simulink model "calcparam1cell"  (R2019a)
settings: Solver=VariableStepAuto  StartTime=0.0  StopTime=2335  RelTol=1e-3
values from neighbouring files (symbols this model uses):
  Q = 31.2    [workspace.mat]
undefined symbols (not defined in the file or in its folder): c1, r0, r1, sigbuilder_block, soc_1
settings Model: Creator=sujan  LastModifiedBy=sujan

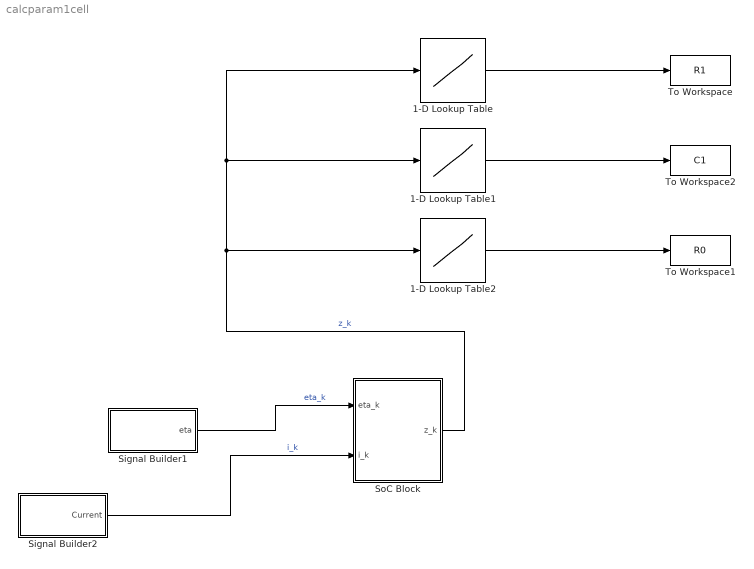
== system calcparam1cell ==
  1-D Lookup Table : Lookup_n-D  NumberOfTableDimensions=1  BreakpointsForDimension1=soc_1.soc_1  Table=r1.r1  InternalRulePriority=Speed  RndMeth=Simplest  InputSameDT=on
  1-D Lookup Table1 : Lookup_n-D  NumberOfTableDimensions=1  BreakpointsForDimension1=soc_1.soc_1  Table=c1.c1  InternalRulePriority=Speed  RndMeth=Simplest  InputSameDT=on
  1-D Lookup Table2 : Lookup_n-D  NumberOfTableDimensions=1  BreakpointsForDimension1=soc_1.soc_1  Table=r0.r0  InternalRulePriority=Speed  RndMeth=Simplest  InputSameDT=on
  Signal Builder1 : Subsystem  Tag=STV Subsys  LoadFcn=sigbuilder_block('load');  StartFcn=sigbuilder_block('start');  StopFcn=sigbuilder_block('stop');  ClipboardFcn=sigbuilder_block('clipboard');  mask(Sigbuilder block){tuvar=[0:10]}
      mask help: Simulink:masks:SigbuilderBlock_MD
      mask init:
      | if ~strcmp(get_param(bdroot(gcbh),'SimulationStatus'),'stopped') tuvar = sigbuilder_block('maskInit'); end
      settings: CopyFcn=sigbuilder_block('copy');  DeleteFcn=sigbuilder_block('delete');  ModelCloseFcn=sigbuilder_block('modelClose');  PreSaveFcn=sigbuilder_block('preSave');  PauseFcn=sigbuilder_block('pause');  ContinueFcn=sigbuilder_block('continue');  NameChangeFcn=sigbuilder_block('namechange');  OpenFcn=sigbuilder_block('open',[402.6 159.6 550.8 400.2 ]);  CloseFcn=sigbuilder_block('close');
      mask Display: plot(0, 0, 100, 100,[2, 2, 32, 32, 2], [68, 8, 8, 68, 68],[32, 2], [38, 38], [32, 19, 2],[53, 60, 44], [32, 17, 17, 2],[16, 16, 31, 31]);txt = getActiveGroup(gcbh);text(2, 100, txt,'verticalAlignment', 'top');
  Signal Builder2 : Subsystem  Tag=STV Subsys  LoadFcn=sigbuilder_block('load');  StartFcn=sigbuilder_block('start');  StopFcn=sigbuilder_block('stop');  ClipboardFcn=sigbuilder_block('clipboard');  mask(Sigbuilder block){tuvar=[0:10]}
      mask help: Simulink:masks:SigbuilderBlock_MD
      mask init:
      | if ~strcmp(get_param(bdroot(gcbh),'SimulationStatus'),'stopped') tuvar = sigbuilder_block('maskInit'); end
      settings: CopyFcn=sigbuilder_block('copy');  DeleteFcn=sigbuilder_block('delete');  ModelCloseFcn=sigbuilder_block('modelClose');  PreSaveFcn=sigbuilder_block('preSave');  PauseFcn=sigbuilder_block('pause');  ContinueFcn=sigbuilder_block('continue');  NameChangeFcn=sigbuilder_block('namechange');  OpenFcn=sigbuilder_block('open',[339.6 151.8 550.8 400.2 ]);  CloseFcn=sigbuilder_block('close');
      mask Display: plot(0, 0, 100, 100,[2, 2, 32, 32, 2], [68, 8, 8, 68, 68],[32, 2], [38, 38], [32, 19, 2],[53, 60, 44], [32, 17, 17, 2],[16, 16, 31, 31]);txt = getActiveGroup(gcbh);text(2, 100, txt,'verticalAlignment', 'top');
  "SoC Block " : Subsystem
  To Workspace : ToWorkspace  VariableName=R1  SaveFormat=Timeseries  SampleTime=-1
      settings: Save2DSignal=2-D array (concatenate along first dimension)
  To Workspace1 : ToWorkspace  VariableName=R0  SaveFormat=Timeseries  SampleTime=-1
      settings: Save2DSignal=2-D array (concatenate along first dimension)
  To Workspace2 : ToWorkspace  VariableName=C1  SaveFormat=Timeseries  SampleTime=-1
      settings: Save2DSignal=2-D array (concatenate along first dimension)
  wires:
  Signal Builder1/1(eta) -> "SoC Block "/1(eta_k)  "eta_k"
  "SoC Block "/1(z_k) -> 1-D Lookup Table/1, 1-D Lookup Table1/1, 1-D Lookup Table2/1  "z_k"
  Signal Builder2/1(Current) -> "SoC Block "/2(i_k)  "i_k"
  1-D Lookup Table1/1 -> To Workspace2/1
  1-D Lookup Table2/1 -> To Workspace1/1
  1-D Lookup Table/1 -> To Workspace/1

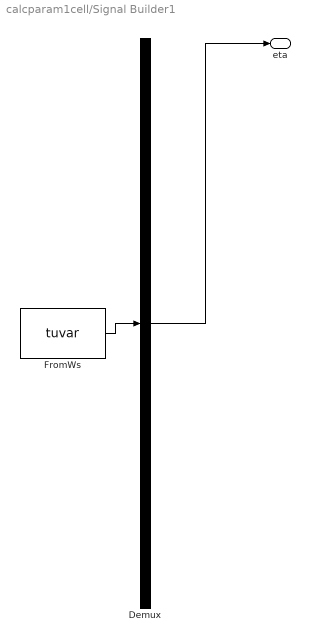
== system calcparam1cell/Signal Builder1 ==
  Demux : Demux  Tag=STV Demux  Outputs=1
  FromWs : FromWorkspace  Tag=STV FromWs  VariableName=tuvar  SampleTime=0
      SigBuilderData=|
      | common.afterFinalStr = 'Extrapolate'
      | common.sampleTime = 0
      | dataSet.timeRange = [0.0176671365608 124.786676059]
      | dataSet.name = 'Sheet1'
      | sbobj.Groups.Name = 'Sheet1'
      | sbobj.Groups.Signals.Name = 'eta'
      | sbobj.Groups.Signals.XData = [0.0176671365608 0.117667136561 0.219171291651 0.303787743842 0.378074200794 0.445155666779 0.506826698763 0.564234547563 0.618167124509 0.669194043835 0.717743348713 0.76414658576 ... (9908 elements, 1x9908)]
      | sbobj.Groups.Signals.YData = [0.954687407395 0.903905741593 0.906290104529 0.908282961266 0.909894745679 0.911352190394 0.91269410615 0.913944970125 0.915121594024 0.916236132604 0.917297720353 0.918313433014 ... (9908 elements, 1x9908)]
      | sbobj.Groups.TimeRange = [0.0176671365608 124.786676059]
  eta : Outport  Tag=STV Outport
  wires:
  Demux/1 -> eta/1
  FromWs/1 -> Demux/1

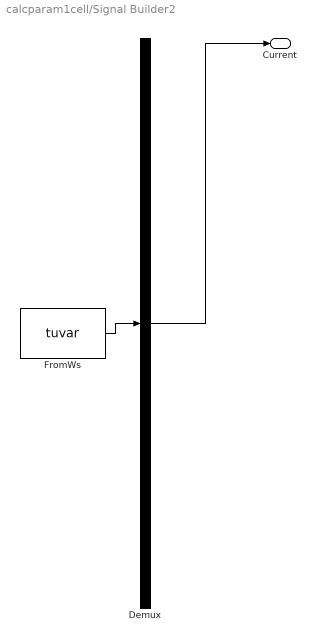
== system calcparam1cell/Signal Builder2 ==
  Demux : Demux  Tag=STV Demux  Outputs=1
  FromWs : FromWorkspace  Tag=STV FromWs  VariableName=tuvar  SampleTime=0
      SigBuilderData=|
      | common.afterFinalStr = 'Extrapolate'
      | common.sampleTime = 0
      | dataSet.timeRange = [0.0176671365608 124.786676059]
      | dataSet.name = 'Sheet1'
      | sbobj.Groups.Name = 'Sheet1'
      | sbobj.Groups.Signals.Name = 'Current'
      | sbobj.Groups.Signals.XData = [0.0176671365608 0.117667136561 0.219171291651 0.303787743842 0.378074200794 0.445155666779 0.506826698763 0.564234547563 0.618167124509 0.669194043835 0.717743348713 0.76414658576 ... (9908 elements, 1x9908)]
      | sbobj.Groups.Signals.YData = [12.5889164833 11.9192877182 11.9507289477 11.977007609 11.9982612876 12.017479777 12.0351748521 12.0516692795 12.0671847455 12.0818815279 12.095880078 12.1092736996 ... (9908 elements, 1x9908)]
      | sbobj.Groups.TimeRange = [0.0176671365608 124.786676059]
  Current : Outport  Tag=STV Outport
  wires:
  Demux/1 -> Current/1
  FromWs/1 -> Demux/1

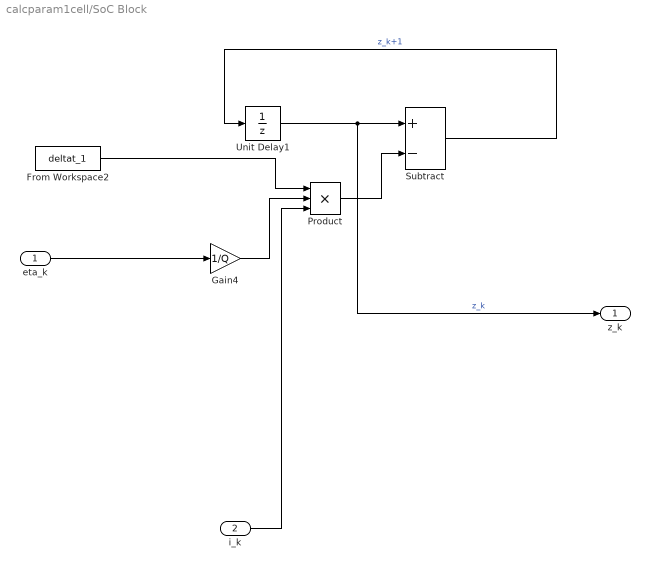
== system calcparam1cell/SoC Block  ==
  eta_k : Inport
  i_k : Inport  Port=2
  From Workspace2 : FromWorkspace  VariableName=deltat_1  SampleTime=0
  Gain4 : Gain  Gain=1/Q
  Product : Product  Inputs=3
  Subtract : Sum  Inputs=+-
  Unit Delay1 : UnitDelay  InitialCondition=100  HasFrameUpgradeWarning=on
  z_k : Outport
  wires:
  Product/1 -> Subtract/2
  From Workspace2/1 -> Product/1
  Unit Delay1/1 -> z_k/1, Subtract/1  "z_k"
  eta_k/1 -> Gain4/1
  Gain4/1 -> Product/2
  i_k/1 -> Product/3
  Subtract/1 -> Unit Delay1/1  "z_k+1"
